simulink model "EoM_TEST1"  (R2016b)
settings: Solver=VariableStepAuto  StartTime=0.0  StopTime=60  RelTol=1e-3
values from neighbouring files (symbols this model uses):
  CG = [0;1;0]    [InitTestBench.m]
  DOWN_0 = 0    [InitTestBench.m]
  EAST_0 = 0    [InitTestBench.m]
  FORCES = [X;Y;Z]    [InitTestBench.m]
  INERTIA = [0 0 0 ... (first row only)    [InitTestBench.m]
  MASS = 1    [InitTestBench.m]
  MOMENTS = [L;M;N]    [InitTestBench.m]
  NORTH_0 = 0    [InitTestBench.m]
  P_0 = 0    [InitTestBench.m]
  PHI_0 = -pi/4    (= -0.785398163397)    [InitTestBench.m]
  PSI_0 = 0    [InitTestBench.m]
  Q_0 = 0    [InitTestBench.m]
  R_0 = 0    [InitTestBench.m]
  THETA_0 = 0    [InitTestBench.m]
  U_0 = 0    [InitTestBench.m]
  V_0 = 0    [InitTestBench.m]
  W_0 = 0    [InitTestBench.m]
settings Model: Creator=pereantoni  LastModifiedBy=carles

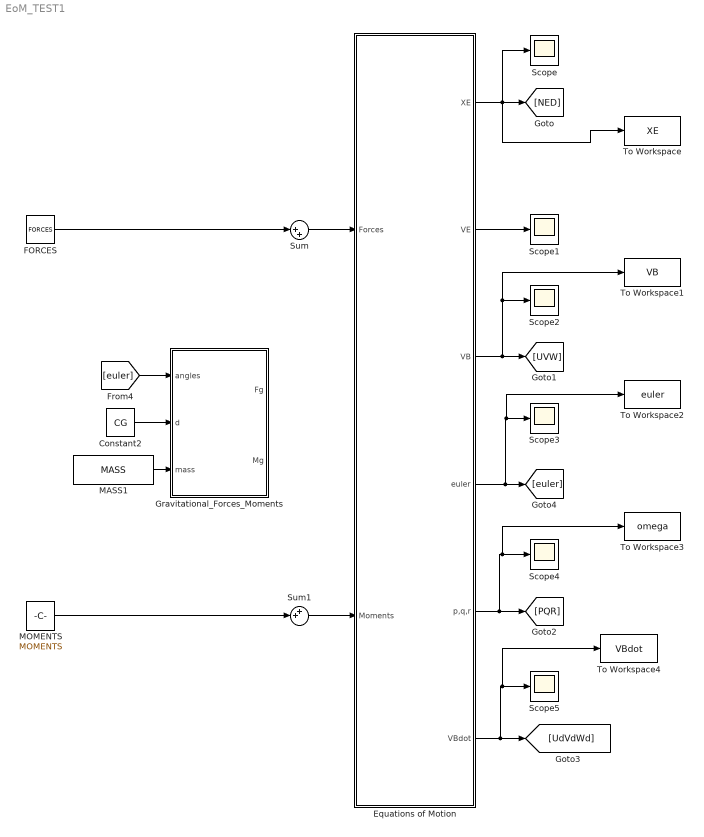
== system EoM_TEST1 ==
  Constant2 : Constant  Value=CG
  Equations of Motion : Subsystem
  FORCES : Constant  Value=FORCES
  Gravitational_Forces_Moments : MATLAB Function  TreatAsAtomicUnit=on
  MASS1 : Constant  Value=MASS
  MOMENTS : Constant  Value=MOMENTS
  Scope{,1..5} (6 alike) : Scope
  Sum : Sum  Inputs=|++
  Sum1 : Sum  Inputs=++|
  To Workspace : ToWorkspace  VariableName=XE  SaveFormat=Timeseries  SampleTime=-1
  To Workspace1 : ToWorkspace  VariableName=VB  SaveFormat=Timeseries  SampleTime=-1
  To Workspace2 : ToWorkspace  VariableName=euler  SaveFormat=Timeseries  SampleTime=-1
  To Workspace3 : ToWorkspace  VariableName=omega  SaveFormat=Timeseries  SampleTime=-1
  To Workspace4 : ToWorkspace  VariableName=VBdot  SaveFormat=Timeseries  SampleTime=-1
  wires:
  Equations of Motion/1(XE) -> To Workspace/1, Scope/1, [NED]
  Equations of Motion/3(VB) -> To Workspace1/1, Scope2/1, [UVW]
  Equations of Motion/4(euler) -> To Workspace2/1, Scope3/1, [euler]
  Equations of Motion/5(p,q,r) -> To Workspace3/1, Scope4/1, [PQR]
  Equations of Motion/6(VBdot) -> To Workspace4/1, Scope5/1, [UdVdWd]
  Constant2/1 -> Gravitational_Forces_Moments/2(d)
  MASS1/1 -> Gravitational_Forces_Moments/3(mass)
  Sum/1 -> Equations of Motion/1(Forces)
  Sum1/1 -> Equations of Motion/2(Moments)
  [euler] -> Gravitational_Forces_Moments/1(angles)
  Equations of Motion/2(VE) -> Scope1/1
  FORCES/1 -> Sum/1
  MOMENTS/1 -> Sum1/2

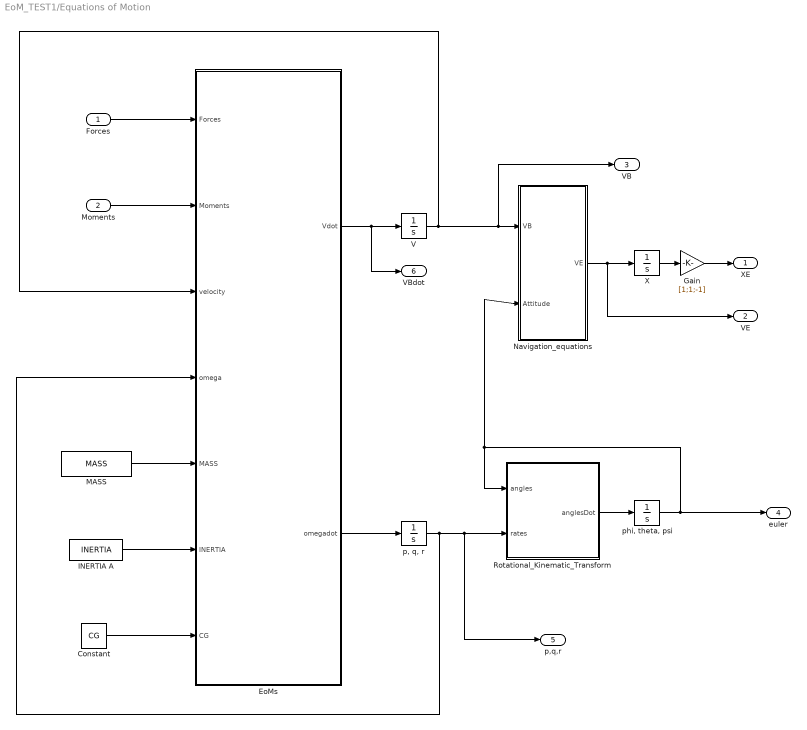
== system EoM_TEST1/Equations of Motion ==
  Forces : Inport
  Moments : Inport  Port=2
  Constant : Constant  Value=CG
  EoMs : MATLAB Function  TreatAsAtomicUnit=on
  Gain : Gain  Gain=[1;1;-1]
  INERTIA A : Constant  Value=INERTIA
  MASS : Constant  Value=MASS
  Navigation_equations : Subsystem
  Rotational_Kinematic_Transform : MATLAB Function  TreatAsAtomicUnit=on
  V : Integrator  Tag='V'  Priority=1  InitialCondition=[U_0;V_0;W_0]  ContinuousStateAttributes='V'
  X : Integrator  Tag='X'  Priority=4  InitialCondition=[NORTH_0 EAST_0 -DOWN_0]  ContinuousStateAttributes='X'
  "p, q, r" : Integrator  Tag='omega'  Priority=2  InitialCondition=[P_0;Q_0;R_0]  ContinuousStateAttributes='omega'
  "phi, theta, psi" : Integrator  Tag='euler'  Priority=3  InitialCondition=[PHI_0;THETA_0;PSI_0]  ContinuousStateAttributes='euler'
  XE : Outport
  VE : Outport  Port=2
  VB : Outport  Port=3
  euler : Outport  Port=4
  p,q,r : Outport  Port=5
  VBdot : Outport  Port=6
  wires:
  INERTIA A/1 -> EoMs/6(INERTIA)
  MASS/1 -> EoMs/5(MASS)
  X/1 -> Gain/1
  V/1 -> Navigation_equations/1(VB), VB/1, EoMs/3(velocity)
  "p, q, r"/1 -> Rotational_Kinematic_Transform/2(rates), p,q,r/1, EoMs/4(omega)
  EoMs/1(Vdot) -> VBdot/1, V/1
  Constant/1 -> EoMs/7(CG)
  Forces/1 -> EoMs/1(Forces)
  Moments/1 -> EoMs/2(Moments)
  EoMs/2(omegadot) -> "p, q, r"/1
  Rotational_Kinematic_Transform/1(anglesDot) -> "phi, theta, psi"/1
  "phi, theta, psi"/1 -> euler/1, Navigation_equations/2(Attitude), Rotational_Kinematic_Transform/1(angles)
  Gain/1 -> XE/1
  Navigation_equations/1(VE) -> VE/1, X/1

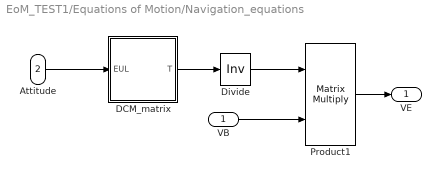
== system EoM_TEST1/Equations of Motion/Navigation_equations ==
  VB : Inport
  Attitude : Inport  Port=2
  DCM_matrix : MATLAB Function  TreatAsAtomicUnit=on
  Divide : Product  Inputs=/  Multiplication=Matrix(*)
  Product1 : Product  Multiplication=Matrix(*)
  VE : Outport
  wires:
  Attitude/1 -> DCM_matrix/1(EUL)
  VB/1 -> Product1/2
  DCM_matrix/1(T) -> Divide/1
  Product1/1 -> VE/1
  Divide/1 -> Product1/1

== matlab function EoM_TEST1/Equations of Motion/Navigation_equations/DCM_matrix ==
  data: EUL input; T output
function T  = DCM(EUL)

%Euler Angles
Phi   = EUL(1);
Theta = EUL(2);
Psi   = EUL(3);

%% Cosine Matrix

T = zeros (3,3);

T(1,1) = cos(Theta)*cos(Psi);
T(1,2) = cos(Theta)*sin(Psi);
T(1,3) = -sin(Theta);

T(2,1) = -cos(Phi)*sin(Psi) + sin(Phi)*sin(Theta)*cos(Psi);
T(2,2) = cos(Phi)*cos(Psi) +sin(Phi)*sin(Theta)*sin(Psi);
T(2,3) = sin(Phi)*cos(Theta);

T(3,1) = sin(Phi)*sin(Psi) + cos(Phi)*sin(Theta)*cos(Psi);
T(3,2) = -sin(Phi)*cos(Psi)+ cos(Phi)*sin(Theta)*sin(Psi);
T(3,3) = cos(Phi)*cos(Theta);
end

== matlab function EoM_TEST1/Equations of Motion/EoMs ==
  data: Forces input; Vdot output; Moments input; velocity input; omega input; omegadot output; MASS input; INERTIA input; CG input
function [Vdot,omegadot]= Equations_of_Motion(Forces,Moments,velocity,omega,MASS,INERTIA,CG)
%Variable definition
m=MASS;
dx=CG(1);
dy=CG(2);
dz=CG(3);
I=INERTIA;
Ixx=I(1,1);
Iyy=I(2,2);
Izz=I(3,3);
Ixz=I(1,3);


U=velocity(1);
V=velocity(2);
W=velocity(3);

P=omega(1);
Q=omega(2);
R=omega(3);


X=Forces(1);
Y=Forces(2);
Z=Forces(3);

L=Moments(1);
M=Moments(2);
N=Moments(3);

% Motion's Matrix composition


massProperties=[
        m       0       0       0       m*dz   -m*dy;
        0       m       0      -m*dz    0       m*dx;
        0       0       m       m*dy   -m*dx    0   ;
        0      -m*dz    m*dy    Ixx     0      -Ixz ;
        m*dz    0      -m*dx    0       Iyy     0   ;
       -m*dy    m*dx    0      -Ixz     0       Izz  ];
   
dynamicProperties=[
        X+m*R*V-m*Q*W+m*dx*(Q^2+R^2)-m*dy*P*Q-m*dz*P*R;
        Y-m*R*U+m*P*W-m*dx*P*Q+m*dy*(P^2+R^2)-m*dz*Q*R;
        Z+m*Q*U-m*P*V-m*dx*P*R+m*dy*Q*R+m*dz*(P^2+Q^2);
        L-Q*R*(Izz-Iyy)+P*Q*Ixz-(P*V-Q*U)*m*dy+(R*U-P*W)*m*dz;
        M-P*R*(Ixx-Izz)-(P^2-R^2)*Ixz-(Q*U-P*V)*m*dx-(Q*W-R*V)*m*dz;
        N-P*Q*(Iyy-Ixx)-Q*R*Ixz-(R*U-P*W)*m*dx+(Q*W-R*V)*m*dy];
 
% Motion output
    
motion=massProperties\dynamicProperties;  


Vdot        =motion(1:3);
omegadot    =motion(4:6);

%Problemes:
%dx in angular

end

== matlab function EoM_TEST1/Equations of Motion/Rotational_Kinematic_Transform ==
  data: angles input; rates input; anglesDot output
function anglesDot   = rotationalkinematic(angles, rates)

phi = angles(1);
theta = angles(2);

P = rates(1);
Q = rates(2);
R = rates(3);

transfMat = [1, sin(phi).*tan(theta), cos(phi).*tan(theta);...
			0, cos(phi), -sin(phi);...
			0, sin(phi).*sec(theta), cos(phi).*sec(theta)];

anglesDot = transfMat*[P; Q; R];

end

== matlab function EoM_TEST1/Gravitational_Forces_Moments ==
  data: angles input; d input; mass input; Fg output; Mg output
function [Fg, Mg] = gravityFn(angles, d, mass)

dx = d(1);
dy = d(2);
dz = d(3);

phi = angles(1);
theta = angles(2);

gMat = [-mass*9.81*sin(theta);
		mass*9.81*sin(phi)*cos(theta);
		mass*9.81*cos(phi)*cos(theta)];

mat = [1, 0, 0;
		0, 1, 0;
		0, 0, 1;
		0, -dz, dy;
		dz, 0, -dx; % it is wrong in the notes, there, the terms are swapped and dx does not have the "minus sign"
		-dy, dx, 0];
    
X = mat*gMat;

Fg = [X(1); X(2); X(3)];
Mg = [X(4); X(5); X(6)];
end
